simulink model "gm_uz_pmsm_model_nonlinear_vnl"  (R2023a)
settings: Solver=FixedStepAuto  StartTime=0.0  StopTime=0.5  RelTol=1e-3
PreLoadFcn:
  | uz_pmsm_model_init_parameter
PostLoadFcn:
  | % Import the data from Excel for a lookup table
  | FluxMapData = readtable('C:\Users\Philipp\ultrazohm\ultrazohm_sw\ip_cores\uz_pmsm_model\FluxMapData_2023-05-26_13-07-57.csv');
  | % Row indices for lookup table
  | d_current_in_d_axis = FluxMapData(8:27,1:end);
  | % Column indices for lookup table
  | q_current_in_d_axis = FluxMapData(29:48,1:end);
  | % Output values for lookup table
  | d_Flux_d_axis = FluxMapData(50:69,1:end);
undefined symbols (not defined in the file or in its folder): d_current_d_Flux, d_current_q_Flux, Flux_d, Flux_q, friction_coefficient, inertia, k_i_d, k_p_d, k_p_q, L_d, L_q, Ldd, Ldq, Lqd, Lqq, polepair, psi_pm, q_current_d_Flux, q_current_q_Flux, R_1, setpoint_step, simulate_mechanical, simulate_open_loop, static_friction_torque, ts
libraries: hdlmdlgenlib x8, simulink x2, slpidlib x2
(part 2 of 2)

== system gm_uz_pmsm_model_nonlinear_vnl/uz_pmsm_model_nonlinear/Divide_recip ==
  In1 : Inport
  Divide_recip : Math  Operator=reciprocal  SampleTime=1e-08
  Divide_recip_pd1 : Delay  DelayLength=30
  Out1 : Outport
  wires:
  Divide_recip_pd1/1 -> Out1/1
  Divide_recip/1 -> Divide_recip_pd1/1
  In1/1 -> Divide_recip/1

== system gm_uz_pmsm_model_nonlinear_vnl/uz_pmsm_model_nonlinear/Factor ==
  In1 : Inport
  In2 : Inport  Port=2
  Factor : Product  Inputs=**  OutDataTypeStr=double  SampleTime=1e-08
  Factor_pd1 : Delay  DelayLength=6
  Out1 : Outport
  wires:
  Factor_pd1/1 -> Out1/1
  Factor/1 -> Factor_pd1/1
  In2/1 -> Factor/2
  In1/1 -> Factor/1

== system gm_uz_pmsm_model_nonlinear_vnl/uz_pmsm_model_nonlinear/Flux_d Lookup Table ==
  In1 : Inport
  In2 : Inport  Port=2
  Flux_d Lookup Table : Lookup_n-D  BreakpointsForDimension1=d_current_d_Flux  BreakpointsForDimension2=q_current_d_Flux  BreakpointsForDimension3=[5, 7]  Table=Flux_d  InternalRulePriority=Speed  RndMeth=Simplest
      settings: InputPortMap=u0,u1
  Flux_d Lookup Table_pd1 : Delay  DelayLength=68
  Out1 : Outport
  wires:
  In1/1 -> Flux_d Lookup Table/1
  Flux_d Lookup Table/1 -> Flux_d Lookup Table_pd1/1
  In2/1 -> Flux_d Lookup Table/2
  Flux_d Lookup Table_pd1/1 -> Out1/1

== system gm_uz_pmsm_model_nonlinear_vnl/uz_pmsm_model_nonlinear/Flux_q Lookup Table ==
  In1 : Inport
  In2 : Inport  Port=2
  Flux_q Lookup Table : Lookup_n-D  BreakpointsForDimension1=d_current_q_Flux  BreakpointsForDimension2=q_current_q_Flux  BreakpointsForDimension3=[5, 7]  Table=Flux_q  InternalRulePriority=Speed  RndMeth=Simplest
      settings: InputPortMap=u0,u1
  Flux_q Lookup Table_pd1 : Delay  DelayLength=68
  Out1 : Outport
  wires:
  In2/1 -> Flux_q Lookup Table/2
  Flux_q Lookup Table/1 -> Flux_q Lookup Table_pd1/1
  Flux_q Lookup Table_pd1/1 -> Out1/1
  In1/1 -> Flux_q Lookup Table/1

== system gm_uz_pmsm_model_nonlinear_vnl/uz_pmsm_model_nonlinear/Gain ==
  In1 : Inport
  In2 : Inport  Port=2
  Gain : Product  Inputs=**  OutDataTypeStr=double  SampleTime=1e-08
  Gain_pd1 : Delay  DelayLength=6
  Out1 : Outport
  wires:
  Gain_pd1/1 -> Out1/1
  Gain/1 -> Gain_pd1/1
  In2/1 -> Gain/2
  In1/1 -> Gain/1

== system gm_uz_pmsm_model_nonlinear_vnl/uz_pmsm_model_nonlinear/Gain7 ==
  In1 : Inport
  In2 : Inport  Port=2
  Gain7 : Product  Inputs=**  OutDataTypeStr=double  SampleTime=1e-08
  Gain7_pd1 : Delay  DelayLength=6
  Out1 : Outport
  wires:
  Gain7_pd1/1 -> Out1/1
  Gain7/1 -> Gain7_pd1/1
  In2/1 -> Gain7/2
  In1/1 -> Gain7/1

== system gm_uz_pmsm_model_nonlinear_vnl/uz_pmsm_model_nonlinear/Gain71 ==
  In1 : Inport
  In2 : Inport  Port=2
  Gain71 : Product  Inputs=**  OutDataTypeStr=double  SampleTime=1e-08
  Gain71_pd1 : Delay  DelayLength=6
  Out1 : Outport
  wires:
  Gain71_pd1/1 -> Out1/1
  Gain71/1 -> Gain71_pd1/1
  In2/1 -> Gain71/2
  In1/1 -> Gain71/1

== system gm_uz_pmsm_model_nonlinear_vnl/uz_pmsm_model_nonlinear/Ldd Lookup Table ==
  In1 : Inport
  In2 : Inport  Port=2
  Ldd Lookup Table : Lookup_n-D  BreakpointsForDimension1=d_current_q_Flux  BreakpointsForDimension2=q_current_q_Flux  BreakpointsForDimension3=[5, 7]  Table=Ldd  InternalRulePriority=Speed  RndMeth=Simplest
      settings: InputPortMap=u0,u1
  Ldd Lookup Table_pd1 : Delay  DelayLength=68
  Out1 : Outport
  wires:
  Ldd Lookup Table/1 -> Ldd Lookup Table_pd1/1
  In2/1 -> Ldd Lookup Table/2
  In1/1 -> Ldd Lookup Table/1
  Ldd Lookup Table_pd1/1 -> Out1/1

== system gm_uz_pmsm_model_nonlinear_vnl/uz_pmsm_model_nonlinear/Ldq Lookup Table2 ==
  In1 : Inport
  In2 : Inport  Port=2
  Ldq Lookup Table2 : Lookup_n-D  BreakpointsForDimension1=d_current_q_Flux  BreakpointsForDimension2=q_current_q_Flux  BreakpointsForDimension3=[5, 7]  Table=Ldq  InternalRulePriority=Speed  RndMeth=Simplest
      settings: InputPortMap=u0,u1
  Ldq Lookup Table2_pd1 : Delay  DelayLength=68
  Out1 : Outport
  wires:
  In2/1 -> Ldq Lookup Table2/2
  In1/1 -> Ldq Lookup Table2/1
  Ldq Lookup Table2/1 -> Ldq Lookup Table2_pd1/1
  Ldq Lookup Table2_pd1/1 -> Out1/1

== system gm_uz_pmsm_model_nonlinear_vnl/uz_pmsm_model_nonlinear/Lqd Lookup Table1 ==
  In1 : Inport
  In2 : Inport  Port=2
  Lqd Lookup Table1 : Lookup_n-D  BreakpointsForDimension1=d_current_q_Flux  BreakpointsForDimension2=q_current_q_Flux  BreakpointsForDimension3=[5, 7]  Table=Lqd  InternalRulePriority=Speed  RndMeth=Simplest
      settings: InputPortMap=u0,u1
  Lqd Lookup Table1_pd1 : Delay  DelayLength=68
  Out1 : Outport
  wires:
  In1/1 -> Lqd Lookup Table1/1
  In2/1 -> Lqd Lookup Table1/2
  Lqd Lookup Table1/1 -> Lqd Lookup Table1_pd1/1
  Lqd Lookup Table1_pd1/1 -> Out1/1

== system gm_uz_pmsm_model_nonlinear_vnl/uz_pmsm_model_nonlinear/Lqq Lookup Table ==
  In1 : Inport
  In2 : Inport  Port=2
  Lqq Lookup Table : Lookup_n-D  BreakpointsForDimension1=d_current_q_Flux  BreakpointsForDimension2=q_current_q_Flux  BreakpointsForDimension3=[5, 7]  Table=Lqq  InternalRulePriority=Speed  RndMeth=Simplest
      settings: InputPortMap=u0,u1
  Lqq Lookup Table_pd1 : Delay  DelayLength=68
  Out1 : Outport
  wires:
  Lqq Lookup Table_pd1/1 -> Out1/1
  Lqq Lookup Table/1 -> Lqq Lookup Table_pd1/1
  In2/1 -> Lqq Lookup Table/2
  In1/1 -> Lqq Lookup Table/1

== system gm_uz_pmsm_model_nonlinear_vnl/uz_pmsm_model_nonlinear/Product11 ==
  In1 : Inport
  In2 : Inport  Port=2
  Product11 : Product  Inputs=**  OutDataTypeStr=double  SampleTime=1e-08
  Product11_pd1 : Delay  DelayLength=6
  Out1 : Outport
  wires:
  Product11_pd1/1 -> Out1/1
  Product11/1 -> Product11_pd1/1
  In2/1 -> Product11/2
  In1/1 -> Product11/1

== system gm_uz_pmsm_model_nonlinear_vnl/uz_pmsm_model_nonlinear/Product111 ==
  In1 : Inport
  In2 : Inport  Port=2
  Product111 : Product  Inputs=**  OutDataTypeStr=double  SampleTime=1e-08
  Product111_pd1 : Delay  DelayLength=6
  Out1 : Outport
  wires:
  Product111_pd1/1 -> Out1/1
  Product111/1 -> Product111_pd1/1
  In2/1 -> Product111/2
  In1/1 -> Product111/1

== system gm_uz_pmsm_model_nonlinear_vnl/uz_pmsm_model_nonlinear/Product12 ==
  In1 : Inport
  In2 : Inport  Port=2
  Product12 : Product  Inputs=**  OutDataTypeStr=double  SampleTime=1e-08
  Product12_pd1 : Delay  DelayLength=6
  Out1 : Outport
  wires:
  Product12_pd1/1 -> Out1/1
  Product12/1 -> Product12_pd1/1
  In2/1 -> Product12/2
  In1/1 -> Product12/1

== system gm_uz_pmsm_model_nonlinear_vnl/uz_pmsm_model_nonlinear/Product121 ==
  In1 : Inport
  In2 : Inport  Port=2
  Product121 : Product  Inputs=**  OutDataTypeStr=double  SampleTime=1e-08
  Product121_pd1 : Delay  DelayLength=6
  Out1 : Outport
  wires:
  Product121_pd1/1 -> Out1/1
  Product121/1 -> Product121_pd1/1
  In2/1 -> Product121/2
  In1/1 -> Product121/1

== system gm_uz_pmsm_model_nonlinear_vnl/uz_pmsm_model_nonlinear/Product13 ==
  In1 : Inport
  In2 : Inport  Port=2
  Product13 : Product  Inputs=**  OutDataTypeStr=double  SampleTime=1e-08
  Product13_pd1 : Delay  DelayLength=6
  Out1 : Outport
  wires:
  Product13_pd1/1 -> Out1/1
  Product13/1 -> Product13_pd1/1
  In2/1 -> Product13/2
  In1/1 -> Product13/1

== system gm_uz_pmsm_model_nonlinear_vnl/uz_pmsm_model_nonlinear/Product2 ==
  In1 : Inport
  In2 : Inport  Port=2
  Product2 : Product  Inputs=**  OutDataTypeStr=double  SampleTime=1e-08
  Product2_pd1 : Delay  DelayLength=6
  Out1 : Outport
  wires:
  Product2_pd1/1 -> Out1/1
  Product2/1 -> Product2_pd1/1
  In2/1 -> Product2/2
  In1/1 -> Product2/1

== system gm_uz_pmsm_model_nonlinear_vnl/uz_pmsm_model_nonlinear/Product21 ==
  In1 : Inport
  In2 : Inport  Port=2
  Product21 : Product  Inputs=**  OutDataTypeStr=double  SampleTime=1e-08
  Product21_pd1 : Delay  DelayLength=6
  Out1 : Outport
  wires:
  Product21_pd1/1 -> Out1/1
  Product21/1 -> Product21_pd1/1
  In2/1 -> Product21/2
  In1/1 -> Product21/1

== system gm_uz_pmsm_model_nonlinear_vnl/uz_pmsm_model_nonlinear/Product3 ==
  In1 : Inport
  In2 : Inport  Port=2
  Product3 : Product  Inputs=**  OutDataTypeStr=double  SampleTime=1e-08
  Product3_pd1 : Delay  DelayLength=6
  Out1 : Outport
  wires:
  Product3_pd1/1 -> Out1/1
  Product3/1 -> Product3_pd1/1
  In2/1 -> Product3/2
  In1/1 -> Product3/1

== system gm_uz_pmsm_model_nonlinear_vnl/uz_pmsm_model_nonlinear/Product31 ==
  In1 : Inport
  In2 : Inport  Port=2
  Product31 : Product  Inputs=**  OutDataTypeStr=double  SampleTime=1e-08
  Product31_pd1 : Delay  DelayLength=6
  Out1 : Outport
  wires:
  Product31_pd1/1 -> Out1/1
  Product31/1 -> Product31_pd1/1
  In2/1 -> Product31/2
  In1/1 -> Product31/1

== system gm_uz_pmsm_model_nonlinear_vnl/uz_pmsm_model_nonlinear/Product4 ==
  In1 : Inport
  In2 : Inport  Port=2
  Product4 : Product  Inputs=**  OutDataTypeStr=double  SampleTime=1e-08
  Product4_pd1 : Delay  DelayLength=6
  Out1 : Outport
  wires:
  Product4_pd1/1 -> Out1/1
  Product4/1 -> Product4_pd1/1
  In2/1 -> Product4/2
  In1/1 -> Product4/1

== system gm_uz_pmsm_model_nonlinear_vnl/uz_pmsm_model_nonlinear/Product41 ==
  In1 : Inport
  In2 : Inport  Port=2
  Product41 : Product  Inputs=**  OutDataTypeStr=double  SampleTime=1e-08
  Product41_pd1 : Delay  DelayLength=6
  Out1 : Outport
  wires:
  Product41_pd1/1 -> Out1/1
  Product41/1 -> Product41_pd1/1
  In2/1 -> Product41/2
  In1/1 -> Product41/1

== system gm_uz_pmsm_model_nonlinear_vnl/uz_pmsm_model_nonlinear/Product9 ==
  In1 : Inport
  In2 : Inport  Port=2
  Product9 : Product  Inputs=**  OutDataTypeStr=double  SampleTime=1e-08
  Product9_pd1 : Delay  DelayLength=6
  Out1 : Outport
  wires:
  Product9_pd1/1 -> Out1/1
  Product9/1 -> Product9_pd1/1
  In2/1 -> Product9/2
  In1/1 -> Product9/1

== system gm_uz_pmsm_model_nonlinear_vnl/uz_pmsm_model_nonlinear/Product91 ==
  In1 : Inport
  In2 : Inport  Port=2
  Product91 : Product  Inputs=**  OutDataTypeStr=double  SampleTime=1e-08
  Product91_pd1 : Delay  DelayLength=6
  Out1 : Outport
  wires:
  Product91_pd1/1 -> Out1/1
  Product91/1 -> Product91_pd1/1
  In2/1 -> Product91/2
  In1/1 -> Product91/1

== system gm_uz_pmsm_model_nonlinear_vnl/uz_pmsm_model_nonlinear/Sign1 ==
  In1 : Inport
  Sign1 : Signum  SampleTime=1e-08
  Out1 : Outport
  wires:
  Sign1/1 -> Out1/1
  In1/1 -> Sign1/1

== system gm_uz_pmsm_model_nonlinear_vnl/uz_pmsm_model_nonlinear/Sum ==
  In1 : Inport
  In2 : Inport  Port=2
  Sum : Sum  Inputs=+-  OutDataTypeStr=double  SampleTime=1e-08
  Sum_pd1 : Delay  DelayLength=6
  Out1 : Outport
  wires:
  Sum_pd1/1 -> Out1/1
  Sum/1 -> Sum_pd1/1
  In2/1 -> Sum/2
  In1/1 -> Sum/1

== system gm_uz_pmsm_model_nonlinear_vnl/uz_pmsm_model_nonlinear/Sum1 ==
  In1 : Inport
  In2 : Inport  Port=2
  Sum1 : Sum  Inputs=+-  OutDataTypeStr=double  SampleTime=1e-08
  Sum1_pd1 : Delay  DelayLength=6
  Out1 : Outport
  wires:
  Sum1_pd1/1 -> Out1/1
  Sum1/1 -> Sum1_pd1/1
  In2/1 -> Sum1/2
  In1/1 -> Sum1/1

== system gm_uz_pmsm_model_nonlinear_vnl/uz_pmsm_model_nonlinear/Sum3 ==
  In1 : Inport
  In2 : Inport  Port=2
  Sum3 : Sum  OutDataTypeStr=double  SampleTime=1e-08
  Sum3_pd1 : Delay  DelayLength=6
  Out1 : Outport
  wires:
  Sum3_pd1/1 -> Out1/1
  Sum3/1 -> Sum3_pd1/1
  In2/1 -> Sum3/2
  In1/1 -> Sum3/1

== system gm_uz_pmsm_model_nonlinear_vnl/uz_pmsm_model_nonlinear/Sum31 ==
  In1 : Inport
  In2 : Inport  Port=2
  Sum31 : Sum  Inputs=+-  OutDataTypeStr=double  SampleTime=1e-08
  Sum31_pd1 : Delay  DelayLength=6
  Out1 : Outport
  wires:
  Sum31_pd1/1 -> Out1/1
  Sum31/1 -> Sum31_pd1/1
  In2/1 -> Sum31/2
  In1/1 -> Sum31/1

== system gm_uz_pmsm_model_nonlinear_vnl/uz_pmsm_model_nonlinear/Sum3_stage2 ==
  In1 : Inport
  In2 : Inport  Port=2
  Sum3_stage2 : Sum  Inputs=+-  OutDataTypeStr=double  SampleTime=1e-08
  Sum3_stage2_pd1 : Delay  DelayLength=6
  Out1 : Outport
  wires:
  Sum3_stage2_pd1/1 -> Out1/1
  Sum3_stage2/1 -> Sum3_stage2_pd1/1
  In2/1 -> Sum3_stage2/2
  In1/1 -> Sum3_stage2/1

== system gm_uz_pmsm_model_nonlinear_vnl/uz_pmsm_model_nonlinear/Sum3_stage3 ==
  In1 : Inport
  In2 : Inport  Port=2
  Sum3_stage3 : Sum  Inputs=+-  OutDataTypeStr=double  SampleTime=1e-08
  Sum3_stage3_pd1 : Delay  DelayLength=6
  Out1 : Outport
  wires:
  Sum3_stage3_pd1/1 -> Out1/1
  Sum3_stage3/1 -> Sum3_stage3_pd1/1
  In2/1 -> Sum3_stage3/2
  In1/1 -> Sum3_stage3/1

== system gm_uz_pmsm_model_nonlinear_vnl/uz_pmsm_model_nonlinear/Sum3_stage4 ==
  In1 : Inport
  In2 : Inport  Port=2
  Sum3_stage4 : Sum  OutDataTypeStr=double  SampleTime=1e-08
  Sum3_stage4_pd1 : Delay  DelayLength=6
  Out1 : Outport
  wires:
  Sum3_stage4_pd1/1 -> Out1/1
  Sum3_stage4/1 -> Sum3_stage4_pd1/1
  In2/1 -> Sum3_stage4/2
  In1/1 -> Sum3_stage4/1

== system gm_uz_pmsm_model_nonlinear_vnl/uz_pmsm_model_nonlinear/Sum4_stage2 ==
  In1 : Inport
  In2 : Inport  Port=2
  Sum4_stage2 : Sum  Inputs=+-  OutDataTypeStr=double  SampleTime=1e-08
  Sum4_stage2_pd1 : Delay  DelayLength=6
  Out1 : Outport
  wires:
  Sum4_stage2_pd1/1 -> Out1/1
  Sum4_stage2/1 -> Sum4_stage2_pd1/1
  In2/1 -> Sum4_stage2/2
  In1/1 -> Sum4_stage2/1

== system gm_uz_pmsm_model_nonlinear_vnl/uz_pmsm_model_nonlinear/Sum4_stage3 ==
  In1 : Inport
  In2 : Inport  Port=2
  Sum4_stage3 : Sum  Inputs=+-  OutDataTypeStr=double  SampleTime=1e-08
  Sum4_stage3_pd1 : Delay  DelayLength=6
  Out1 : Outport
  wires:
  Sum4_stage3_pd1/1 -> Out1/1
  Sum4_stage3/1 -> Sum4_stage3_pd1/1
  In2/1 -> Sum4_stage3/2
  In1/1 -> Sum4_stage3/1

== system gm_uz_pmsm_model_nonlinear_vnl/uz_pmsm_model_nonlinear/Sum4_stage4 ==
  In1 : Inport
  In2 : Inport  Port=2
  Sum4_stage4 : Sum  Inputs=+-  OutDataTypeStr=double  SampleTime=1e-08
  Sum4_stage4_pd1 : Delay  DelayLength=6
  Out1 : Outport
  wires:
  Sum4_stage4_pd1/1 -> Out1/1
  Sum4_stage4/1 -> Sum4_stage4_pd1/1
  In2/1 -> Sum4_stage4/2
  In1/1 -> Sum4_stage4/1

== system gm_uz_pmsm_model_nonlinear_vnl/uz_pmsm_model_nonlinear/Sum5 ==
  In1 : Inport
  In2 : Inport  Port=2
  Sum5 : Sum  OutDataTypeStr=double  SampleTime=1e-08
  Sum5_pd1 : Delay  DelayLength=6
  Out1 : Outport
  wires:
  Sum5_pd1/1 -> Out1/1
  Sum5/1 -> Sum5_pd1/1
  In2/1 -> Sum5/2
  In1/1 -> Sum5/1

== system gm_uz_pmsm_model_nonlinear_vnl/uz_pmsm_model_nonlinear/Sum51 ==
  In1 : Inport
  In2 : Inport  Port=2
  Sum51 : Sum  OutDataTypeStr=double  SampleTime=1e-08
  Sum51_pd1 : Delay  DelayLength=6
  Out1 : Outport
  wires:
  Sum51_pd1/1 -> Out1/1
  Sum51/1 -> Sum51_pd1/1
  In2/1 -> Sum51/2
  In1/1 -> Sum51/1

== system gm_uz_pmsm_model_nonlinear_vnl/uz_pmsm_model_nonlinear/Sum52 ==
  In1 : Inport
  In2 : Inport  Port=2
  Sum52 : Sum  OutDataTypeStr=double  SampleTime=1e-08
  Sum52_pd1 : Delay  DelayLength=6
  Out1 : Outport
  wires:
  Sum52_pd1/1 -> Out1/1
  Sum52/1 -> Sum52_pd1/1
  In2/1 -> Sum52/2
  In1/1 -> Sum52/1

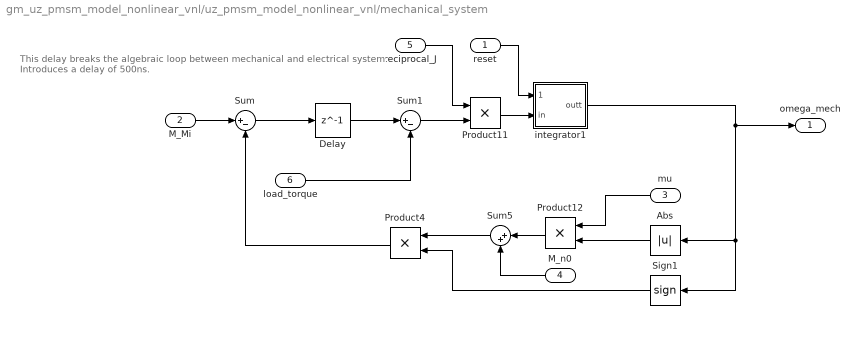
== system gm_uz_pmsm_model_nonlinear_vnl/uz_pmsm_model_nonlinear_vnl/mechanical_system ==
  note: This delay breaks the algebraic loop between mechanical and electrical system.
      | Introduces a delay of 500ns.
  reset : Inport
  M_Mi : Inport  Port=2
  mu : Inport  Port=3
  M_n0 : Inport  Port=4
  reciprocal_J : Inport  Port=5
  load_torque : Inport  Port=6
  Abs : Abs  SaturateOnIntegerOverflow=off
  Delay : Delay  DelayLength=1
  Product11 : Product
  Product12 : Product
  Product4 : Product
  Sign1 : Signum
  Sum : Sum  Inputs=|+-
  Sum1 : Sum  Inputs=|+-
  Sum5 : Sum  Inputs=|++
  integrator1 : Subsystem
  omega_mech : Outport
  wires:
  Delay/1 -> Sum1/1
  Product4/1 -> Sum/2
  Sum/1 -> Delay/1
  load_torque/1 -> Sum1/2
  Sum1/1 -> Product11/2
  M_Mi/1 -> Sum/1
  reciprocal_J/1 -> Product11/1
  M_n0/1 -> Sum5/2
  mu/1 -> Product12/1
  Product12/1 -> Sum5/1
  reset/1 -> integrator1/1(reset)
  Abs/1 -> Product12/2
  integrator1/1(outt) -> omega_mech/1, Abs/1, Sign1/1
  Sign1/1 -> Product4/2
  Sum5/1 -> Product4/1
  Product11/1 -> integrator1/2(in)

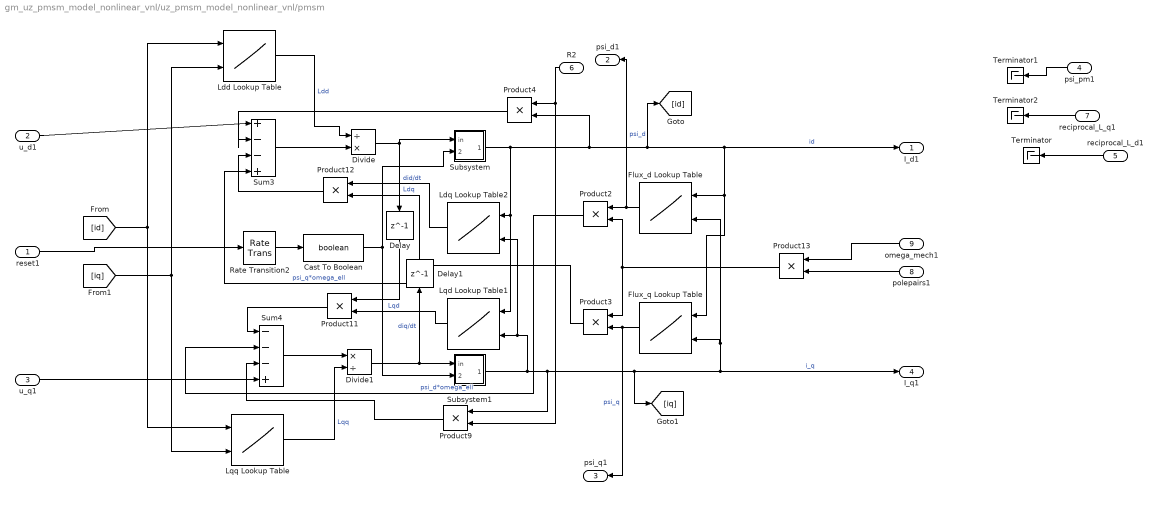
== system gm_uz_pmsm_model_nonlinear_vnl/uz_pmsm_model_nonlinear_vnl/pmsm ==
  reset1 : Inport
  u_d1 : Inport  Port=2
  u_q1 : Inport  Port=3
  psi_pm1 : Inport  Port=4
  reciprocal_L_d1 : Inport  Port=5
  R2 : Inport  Port=6
  reciprocal_L_q1 : Inport  Port=7
  polepairs1 : Inport  Port=8
  omega_mech1 : Inport  Port=9
  Cast To Boolean : DataTypeConversion  OutDataTypeStr=boolean  SaturateOnIntegerOverflow=off  RndMeth=Floor
  Delay : Delay  DelayLength=1
  Delay1 : Delay  DelayLength=1
  Divide : Product  Inputs=/*
  Divide1 : Product  Inputs=*/
  Flux_d Lookup Table : Lookup_n-D  BreakpointsForDimension1=d_current_d_Flux  BreakpointsForDimension2=q_current_d_Flux  BreakpointsForDimension3=[5, 7]  Table=Flux_d  InternalRulePriority=Speed  RndMeth=Simplest
      settings: InputPortMap=u0,u1
  Flux_q Lookup Table : Lookup_n-D  BreakpointsForDimension1=d_current_q_Flux  BreakpointsForDimension2=q_current_q_Flux  BreakpointsForDimension3=[5, 7]  Table=Flux_q  InternalRulePriority=Speed  RndMeth=Simplest
      settings: InputPortMap=u0,u1
  Ldd Lookup Table : Lookup_n-D  BreakpointsForDimension1=d_current_q_Flux  BreakpointsForDimension2=q_current_q_Flux  BreakpointsForDimension3=[5, 7]  Table=Ldd  InternalRulePriority=Speed  RndMeth=Simplest
      settings: InputPortMap=u0,u1
  Ldq Lookup Table2 : Lookup_n-D  BreakpointsForDimension1=d_current_q_Flux  BreakpointsForDimension2=q_current_q_Flux  BreakpointsForDimension3=[5, 7]  Table=Ldq  InternalRulePriority=Speed  RndMeth=Simplest
      settings: InputPortMap=u0,u1
  Lqd Lookup Table1 : Lookup_n-D  BreakpointsForDimension1=d_current_q_Flux  BreakpointsForDimension2=q_current_q_Flux  BreakpointsForDimension3=[5, 7]  Table=Lqd  InternalRulePriority=Speed  RndMeth=Simplest
      settings: InputPortMap=u0,u1
  Lqq Lookup Table : Lookup_n-D  BreakpointsForDimension1=d_current_q_Flux  BreakpointsForDimension2=q_current_q_Flux  BreakpointsForDimension3=[5, 7]  Table=Lqq  InternalRulePriority=Speed  RndMeth=Simplest
      settings: InputPortMap=u0,u1
  Product{2..4,9,11..13} (7 alike) : Product
  Rate Transition2 : RateTransition  OutPortSampleTime=ts
  Subsystem : Subsystem
  Subsystem1 : Subsystem
  Sum3 : Sum  Inputs=|+--+
  Sum4 : Sum  Inputs=|---+
  Terminator : Terminator
  Terminator1 : Terminator
  Terminator2 : Terminator
  I_d1 : Outport
  psi_d1 : Outport  Port=2
  psi_q1 : Outport  Port=3
  I_q1 : Outport  Port=4
  wires:
  Delay1/1 -> Product12/2
  Delay/1 -> Product11/1
  Product2/1 -> Sum4/2  "psi_d*omega_ell"
  Product4/1 -> Sum3/2
  Lqq Lookup Table/1 -> Divide1/2  "Lqq"
  Product3/1 -> Sum3/4  "psi_q*omega_ell"
  Flux_q Lookup Table/1 -> Product3/2, psi_q1/1  "psi_q"
  [iq] -> Lqq Lookup Table/2, Ldd Lookup Table/2
  Subsystem1/1(outt) -> Flux_d Lookup Table/2, Flux_q Lookup Table/2, I_q1/1, [iq], Product9/1, Lqd Lookup Table1/2, Ldq Lookup Table2/2  "i_q"
  psi_pm1/1 -> Terminator1/1
  Ldd Lookup Table/1 -> Divide/1  "Ldd"
  [id] -> Ldd Lookup Table/1, Lqq Lookup Table/1
  Subsystem/1(outt) -> [id], Flux_q Lookup Table/1, Flux_d Lookup Table/1, I_d1/1, Product4/2, Lqd Lookup Table1/1, Ldq Lookup Table2/1  "id"
  R2/1 -> Product4/1, Product9/2
  Rate Transition2/1 -> Cast To Boolean/1
  reciprocal_L_q1/1 -> Terminator2/1
  Product11/1 -> Sum4/1
  reset1/1 -> Rate Transition2/1
  u_d1/1 -> Sum3/1
  Cast To Boolean/1 -> Subsystem1/2(reset), Subsystem/2(reset)
  Product9/1 -> Sum4/3
  Sum3/1 -> Divide/2
  Divide/1 -> Subsystem/1(in), Delay/1  "did/dt"
  Product12/1 -> Sum3/3
  Flux_d Lookup Table/1 -> Product2/1, psi_d1/1  "psi_d"
  Product13/1 -> Product3/1, Product2/2
  Lqd Lookup Table1/1 -> Product11/2  "Lqd"
  polepairs1/1 -> Product13/2
  Divide1/1 -> Delay1/1, Subsystem1/1(in)  "diq/dt"
  reciprocal_L_d1/1 -> Terminator/1
  omega_mech1/1 -> Product13/1
  u_q1/1 -> Sum4/4
  Sum4/1 -> Divide1/1
  Ldq Lookup Table2/1 -> Product12/1  "Ldq"

== system gm_uz_pmsm_model_nonlinear_vnl/uz_pmsm_model_nonlinear_vnl/torque_calculation ==
  I_d : Inport
  psi_d : Inport  Port=2
  psi_q : Inport  Port=3
  polepairs : Inport  Port=4
  I_q : Inport  Port=5
  Factor : Gain  Gain=(3/2)
  Product2 : Product
  Product3 : Product
  Product9 : Product
  Sum3 : Sum  Inputs=-|+
  M_Mi : Outport
  wires:
  Factor/1 -> Product9/1  "M_Mi"
  polepairs/1 -> Product9/2
  Product9/1 -> M_Mi/1  "M_Mi"
  I_q/1 -> Product3/2
  I_d/1 -> Product2/1
  psi_d/1 -> Product3/1
  psi_q/1 -> Product2/2
  Product2/1 -> Sum3/1
  Product3/1 -> Sum3/2
  Sum3/1 -> Factor/1

== system gm_uz_pmsm_model_nonlinear_vnl/Compare/Assert_outputs/RelErrCheck ==
  In1 : Inport
  In2 : Inport  Port=2
  "RelativeErrorCheck " : MATLAB Function  TreatAsAtomicUnit=on
  Out1 : Outport  VectorParamsAs1DForOutWhenUnconnected=off
  wires:
  "RelativeErrorCheck "/1(y) -> Out1/1
  In1/1 -> "RelativeErrorCheck "/1(P)
  In2/1 -> "RelativeErrorCheck "/2(R)

== system gm_uz_pmsm_model_nonlinear_vnl/uz_pmsm_model_nonlinear_vnl/mechanical_system/integrator1 ==
  reset : Inport
  in : Inport  Port=2
  Delay1 : Delay  DelayLength=1  ExternalReset=Level
      settings: InputPortMap=u0,r5
  Gain : Gain  Gain=ts  OutDataTypeStr=double
  Sum3 : Sum  Inputs=|++  OutDataTypeStr=double
  outt : Outport
  wires:
  Delay1/1 -> outt/1, Sum3/2
  Sum3/1 -> Delay1/1
  reset/1 -> Delay1/2
  Gain/1 -> Sum3/1
  in/1 -> Gain/1

== system gm_uz_pmsm_model_nonlinear_vnl/uz_pmsm_model_nonlinear_vnl/pmsm/Subsystem ==
  in : Inport
  reset : Inport  Port=2
  Delay1 : Delay  DelayLength=1  ExternalReset=Level
      settings: InputPortMap=u0,r5
  Gain7 : Gain  Gain=ts  OutDataTypeStr=double
  Sum5 : Sum  Inputs=|++  OutDataTypeStr=double
  outt : Outport
  wires:
  Sum5/1 -> Delay1/1
  Gain7/1 -> Sum5/1
  Delay1/1 -> Sum5/2, outt/1
  reset/1 -> Delay1/2
  in/1 -> Gain7/1

== system gm_uz_pmsm_model_nonlinear_vnl/uz_pmsm_model_nonlinear_vnl/pmsm/Subsystem1 ==
  in : Inport
  reset : Inport  Port=2
  Delay1 : Delay  DelayLength=1  ExternalReset=Level
      settings: InputPortMap=u0,r5
  Gain7 : Gain  Gain=ts  OutDataTypeStr=double
  Sum5 : Sum  Inputs=|++  OutDataTypeStr=double
  outt : Outport
  wires:
  Sum5/1 -> Delay1/1
  Gain7/1 -> Sum5/1
  Delay1/1 -> Sum5/2, outt/1
  reset/1 -> Delay1/2
  in/1 -> Gain7/1

== matlab function gm_uz_pmsm_model_nonlinear_vnl/Compare/Assert_outputs/RelErrCheck/RelativeErrorCheck  ==
  data: P input; y output; R input; ToleranceValue parameter double
% Check if the relative error of R with respect to P is below
% ToleranceValue
% P, R are floating-point
function y = relErrCheck(P,R, ToleranceValue)
    tol = ToleranceValue;
    sz = numel(P);
    assert(sz == numel(R), 'Inputs P and R have different sizes.');
    y = false(1, sz);

    for ii=1:sz
        if (isnan(P(ii)) || isnan(R(ii)))
            if (isnan(P(ii)) && isnan(R(ii)))
                y(ii) = true;
            end
        elseif (isinf(P(ii)) || isinf(R(ii)))
            y(ii) = (P(ii) == R(ii));
        elseif (P(ii) == 0)
            y(ii) = (R(ii) == 0);
        else
            absdiff = abs(P(ii) - R(ii));
            relerr = absdiff/abs(P(ii));
            y(ii) = (relerr <= tol);
        end
    end
end
